simulink model "Bremsdynamik_V1"  (R2016a)
settings: Solver=ode4  StartTime=0.0  StopTime=100  FixedStep=0.0001  RelTol=1e-3
undefined symbols (not defined in the file): A, cW, g, Jr, m, mu, rho, rRad, s, v0
libraries: simulink x1
settings Model: Creator=Michaél  LastModifiedBy=Michaél

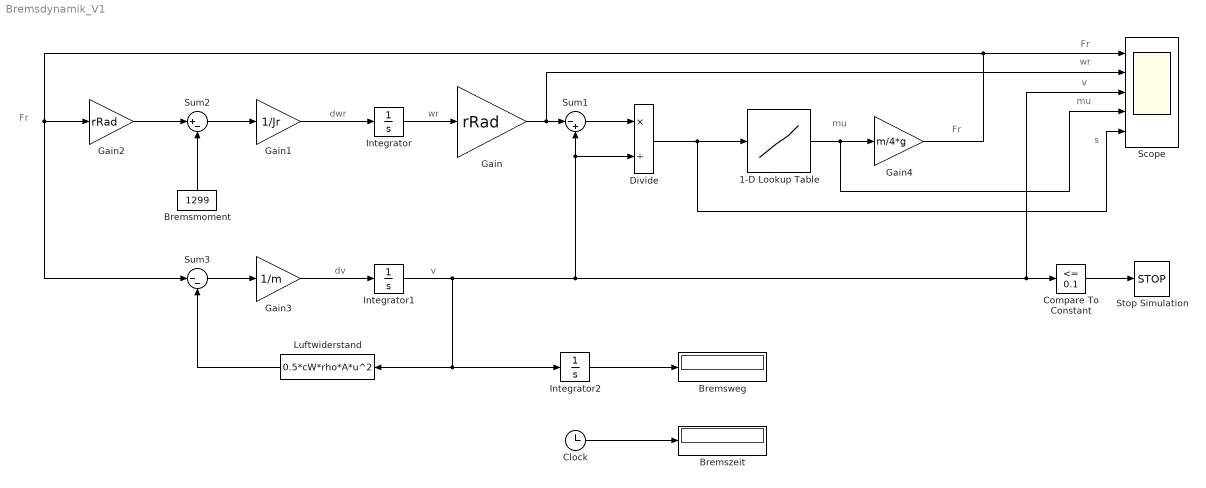
== system Bremsdynamik_V1 ==
  note: s
  note: mu
  note: mu
  note: v
  note: wr
  note: Fr
  note: Fr
  note: Fr
  note: v
  note: dv
  note: dwr
  note: wr
  1-D Lookup Table : Lookup_n-D  NumberOfTableDimensions=1  BreakpointsForDimension1=s  Table=mu  InternalRulePriority=Speed  RndMeth=Simplest  InputSameDT=on
  Bremsmoment : Constant  Value=1299
  Bremsweg : Display
  Bremszeit : Display
  Clock : Clock
  Compare To Constant : simulink/Logic and Bit Operations/Compare To Constant  relop=<=  const=0.1  OutDataTypeStr=boolean
  Divide : Product  Inputs=*/
  Gain : Gain  Gain=rRad
  Gain1 : Gain  Gain=1/Jr
  Gain2 : Gain  Gain=rRad
  Gain3 : Gain  Gain=1/m
  Gain4 : Gain  Gain=m/4*g
  Integrator : Integrator  InitialCondition=v0/rRad  LimitOutput=on  LowerSaturationLimit=0
  Integrator1 : Integrator  InitialCondition=v0  LowerSaturationLimit=0
  Integrator2 : Integrator
  Luftwiderstand : Fcn  Expr=0.5*cW*rho*A*u^2
  Scope : Scope  NumInputPorts=5
  Stop Simulation : Stop
  Sum1 : Sum  Inputs=|-+
  Sum2 : Sum  Inputs=|+-
  Sum3 : Sum  Inputs=|--
  wires:
  Integrator/1 -> Gain/1
  Gain/1 -> Scope/2, Sum1/1
  Sum1/1 -> Divide/1
  Divide/1 -> Scope/5, 1-D Lookup Table/1
  Gain4/1 -> Sum3/1, Gain2/1, Scope/1
  Gain1/1 -> Integrator/1
  Sum2/1 -> Gain1/1
  Gain2/1 -> Sum2/1
  Sum3/1 -> Gain3/1
  Gain3/1 -> Integrator1/1
  Integrator1/1 -> Integrator2/1, Luftwiderstand/1, Scope/3, Compare To Constant/1, Sum1/2, Divide/2
  Luftwiderstand/1 -> Sum3/2
  1-D Lookup Table/1 -> Scope/4, Gain4/1
  Bremsmoment/1 -> Sum2/2
  Compare To Constant/1 -> Stop Simulation/1
  Clock/1 -> Bremszeit/1
  Integrator2/1 -> Bremsweg/1
